simulink model "KD_cl_harness_cl_ouports_added"  (R2015b)
settings: Solver=ode45  StartTime=0  StopTime=inf  FixedStep=0.01  MaxStep=0.005  RelTol=1e-5  AbsTol=1e-5
undefined symbols (not defined in the file or in its folder): A2, bin_vec, c_0, c_1000, c_1000inv, c_100inv, c_1d2p4, c_1p7, c_4400inv, c_5500inv, c_80, c_compmap, c_ctok, c_fflow_max, c_fflow_min, c_filt, c_flowdiv, c_flowmin, c_flowmult, c_inf, c_km1d2k, c_n1, c_p00001, c_p01, c_p1e9, c_p4d1p4, c_pincomp, c_rair, c_roacorr, c_rpmtoradpers, c_svrthrottle1, c_svrthrottle2, c_svrthrottlearg, c_svrthrottlebeta, c_vnliftmax, c_vnliftmin, cl_offset, clff, Coefs, const, const_exhat, const_vec, Dual_array, dual_zero, egr_ecu_ff, expcon, f_mat, gs_jul, HQP_eps, HQP_INF, HQP_saturation, IV, L2, length_L, maxL, mHQP_saturation, minL, Newton, nRed, num_constraints ... (+22)
libraries: simulink x33
(part 5 of 6)

== system KD_cl_harness_cl_ouports_added/ctrl_rb_explicit_20140220_v6_simp/ntremap/remap_wt_to_map/ThrottleModel1/AirModel_map_use ==
  TA_deg : Inport
  Ne_rpm : Inport  Port=2
  Pim_Pa : Inport  Port=3
  Ta_K : Inport  Port=4
  R_a : Inport  Port=5
  wegrthr : Inport  Port=6
  Forward_Flow : Subsystem
  Product1 : Product  Inputs=*//  SaturateOnIntegerOverflow=on  RndMeth=Zero  InputSameDT=on  OutDataTypeStr=Inherit: Same as first input
  Saturation1 : Saturate  UpperLimit=c_inf  LowerLimit=c_p1e9
      settings: AttributesFormatString=%<LowerLimit>\n%<UpperLimit>
  Saturation5 : Saturate  UpperLimit=c_inf  LowerLimit=c_p1e9
      settings: AttributesFormatString=%<LowerLimit>\n%<UpperLimit>
  one : Constant  OutDataTypeStr=single  SampleTime=-1
      settings: AttributesFormatString=%<Value>\n%<SampleTime>
  p_pre_throttle : Outport
  sat_out-45 : Outport  Port=2
  sat_out-46 : Outport  Port=3
  sat_out-58 : Outport  Port=4
  sat_out-59 : Outport  Port=5
  sat_out-60 : Outport  Port=6
  sat_out-61 : Outport  Port=7
  sat_out-62 : Outport  Port=8
  sat_out-63 : Outport  Port=9
  sat_out-64 : Outport  Port=10
  sat_out-65 : Outport  Port=11
  out-17 : Outport  Port=12
  out-28 : Outport  Port=13
  wires:
  Saturation1/1 -> Product1/3
  Saturation5/1 -> Product1/2
  Forward_Flow/1(p_pre_throttle) -> p_pre_throttle/1
  wegrthr/1 -> Forward_Flow/5(wegrthr)
  Ne_rpm/1 -> Forward_Flow/3(Ne_rpm)
  one/1 -> Product1/1
  R_a/1 -> Saturation1/1, sat_out-45/1
  Ta_K/1 -> Saturation5/1, sat_out-46/1
  Pim_Pa/1 -> Forward_Flow/4(Pm)
  TA_deg/1 -> Forward_Flow/2(TA_deg)
  Product1/1 -> Forward_Flow/1(Ro_a)
  Forward_Flow/2(sat_out-58) -> sat_out-58/1
  Forward_Flow/3(sat_out-59) -> sat_out-59/1
  Forward_Flow/4(sat_out-60) -> sat_out-60/1
  Forward_Flow/5(sat_out-61) -> sat_out-61/1
  Forward_Flow/6(sat_out-62) -> sat_out-62/1
  Forward_Flow/7(sat_out-63) -> sat_out-63/1
  Forward_Flow/8(sat_out-64) -> sat_out-64/1
  Forward_Flow/9(sat_out-65) -> sat_out-65/1
  Forward_Flow/10(out-17) -> out-17/1
  Forward_Flow/11(out-28) -> out-28/1

== system KD_cl_harness_cl_ouports_added/ctrl_rb_explicit_20140220_v6_simp/pex_estimator/WhileIteratorSubsystem/newton/For_Iterator_Subsystem ==
  u : Inport
  sv1 : Inport  Port=2
  sv2 : Inport  Port=3
  arg : Inport  Port=4
  beta : Inport  Port=5
  Demux : Demux  Outputs=2
  Divide : Product  Inputs=*/
  For Iterator : ForIterator  ResetStates=reset  IterationLimit=SVR_EGR_exhat.num_SV
  Gain : Gain  Gain=100
      settings: AttributesFormatString=%<Gain>
  Product{,1..3} (4 alike) : Product  RndMeth=Zero
  Saturation1 : Saturate  UpperLimit=9  LowerLimit=1
      settings: AttributesFormatString=%<LowerLimit>\n%<UpperLimit>
  Selector : Selector  InputPortWidth=SVR_EGR_exhat.num_SV  IndexOptions=Index vector (port)  Indices=[1 3]  OutputSizes=1
  Selector1 : Selector  InputPortWidth=SVR_EGR_exhat.num_SV  IndexOptions=Index vector (port)  Indices=[1 3]  OutputSizes=1
  Selector2 : Selector  InputPortWidth=SVR_EGR_exhat.num_SV  IndexOptions=Index vector (port)  Indices=[1 3]  OutputSizes=1
  Sum : Sum  Inputs=|-+
  Sum1 : Sum  Inputs=+-|
  Sum2 : Sum  Inputs=-|-
  Sum3 : Sum  Inputs=++|
  Unit Delay : UnitDelay  SampleTime=-1
  exp Lookup Table : Lookup  InputValues=SVR_EGR_exhat.exp.x  Table=SVR_EGR_exhat.exp.y  LookUpMeth=Interpolation-Use End Values
      settings: AttributesFormatString=%<LookUpMeth>\n%<InputValues>
  ba : Outport  OutDataTypeStr=single
  sat_out-47 : Outport  Port=2
  wires:
  Saturation1/1 -> [iter]
  For Iterator/1 -> Saturation1/1, sat_out-47/1
  [iter] -> Selector2/2
  [iter] -> Selector1/2
  [iter] -> Selector/2
  Sum3/1 -> ba/1, Unit Delay/1
  Product3/1 -> Sum3/2
  Selector2/1 -> Product3/2
  Gain/1 -> Divide/2
  Product2/1 -> Gain/1
  arg/1 -> Product2/2, Product2/1
  Sum2/1 -> Divide/1
  Product1/1 -> Sum2/2
  Product/1 -> Sum2/1
  Sum1/1 -> Product1/2, Product1/1
  Sum/1 -> Product/2, Product/1
  Demux/2 -> Sum1/1
  Selector1/1 -> Sum1/2
  Demux/1 -> Sum/2
  Selector/1 -> Sum/1
  u/1 -> Demux/1
  beta/1 -> Selector2/1
  sv2/1 -> Selector1/1
  sv1/1 -> Selector/1
  Unit Delay/1 -> Sum3/1
  Divide/1 -> exp Lookup Table/1
  exp Lookup Table/1 -> Product3/1

== system KD_cl_harness_cl_ouports_added/ctrl_rb_explicit_20140220_v6_simp/pex_estimator/WhileIteratorSubsystem/newton/If_Action_Subsystem ==
  pex : Inport
  ba : Inport  Port=2
  c : Inport  Port=3
  k : Inport  Port=4
  Action Port : ActionPort  ActionType=then
  Gain1 : Gain  Gain=2
  Gain6 : Gain  Gain=2
  Mux : Mux  Inputs=2
  Product : Product  Inputs=***  RndMeth=Zero
  Product1 : Product  Inputs=*/  RndMeth=Zero
  Product2 : Product  Inputs=**  RndMeth=Zero
  Product3 : Product  Inputs=***  RndMeth=Zero
  Product4 : Product  Inputs=*/  RndMeth=Zero
  Saturation1 : Saturate  UpperLimit=inf  LowerLimit=0
      settings: AttributesFormatString=%<LowerLimit>\n%<UpperLimit>
  Saturation2 : Saturate  UpperLimit=inf  LowerLimit=0
      settings: AttributesFormatString=%<LowerLimit>\n%<UpperLimit>
  Saturation3 : Saturate  UpperLimit=c_inf  LowerLimit=c_p1e9
      settings: AttributesFormatString=%<LowerLimit>\n%<UpperLimit>
  Saturation4 : Saturate  UpperLimit=c_inf  LowerLimit=c_p1e9
      settings: AttributesFormatString=%<LowerLimit>\n%<UpperLimit>
  Sqrt1 : Sqrt  AlgorithmType=Newton-Raphson  SaturateOnIntegerOverflow=on
  Sqrt2 : Sqrt  AlgorithmType=Newton-Raphson  SaturateOnIntegerOverflow=on
  Sum1 : Sum  Inputs=++|
  Sum3 : Sum  Inputs=++|
  one : Constant  OutDataTypeStr=single  SampleTime=-1
      settings: AttributesFormatString=%<Value>\n%<SampleTime>
  one1 : Constant  OutDataTypeStr=single  SampleTime=-1
      settings: AttributesFormatString=%<Value>\n%<SampleTime>
  Out : Outport
  sat_out-48 : Outport  Port=2
  sat_out-49 : Outport  Port=3
  sat_out-50 : Outport  Port=4
  sat_out-51 : Outport  Port=5
  wires:
  Saturation4/1 -> Product4/2
  Saturation3/1 -> Product1/2
  Saturation2/1 -> Sqrt1/1
  Saturation1/1 -> Sqrt2/1
  Product3/1 -> Product2/1
  Sqrt1/1 -> Product3/3
  Product4/1 -> Saturation2/1, sat_out-49/1
  Gain1/1 -> Saturation4/1, sat_out-51/1
  Sum1/1 -> Gain1/1
  one1/1 -> Sum1/1
  [k] -> Sum1/2
  [k] -> Product4/1
  [c] -> Product3/2
  [ba] -> Product3/1
  Mux/1 -> Out/1
  Product2/1 -> Mux/2
  Product/1 -> Mux/1
  Sqrt2/1 -> Product/3
  [pex] -> Product2/2
  Product1/1 -> Saturation1/1, sat_out-48/1
  Gain6/1 -> Saturation3/1, sat_out-50/1
  Sum3/1 -> Gain6/1
  one/1 -> Sum3/1
  [k] -> Sum3/2
  [k] -> Product1/1
  [c] -> Product/2
  [ba] -> Product/1
  k/1 -> [k]
  pex/1 -> [pex]
  c/1 -> [c]
  ba/1 -> [ba]

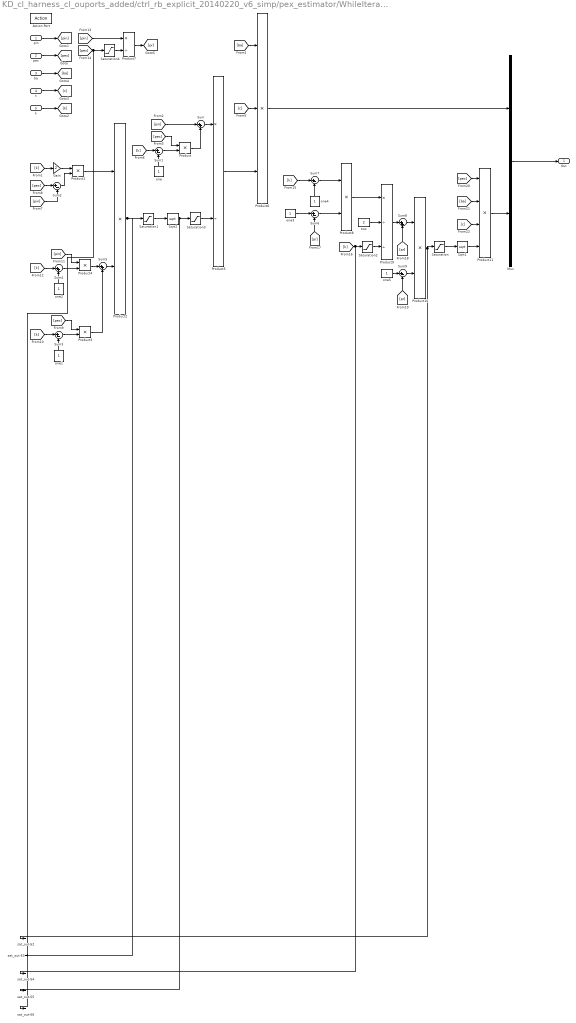
== system KD_cl_harness_cl_ouports_added/ctrl_rb_explicit_20140220_v6_simp/pex_estimator/WhileIteratorSubsystem/newton/If_Action_Subsystem1 ==
  pin : Inport
  pex : Inport  Port=2
  ba : Inport  Port=3
  c : Inport  Port=4
  k : Inport  Port=5
  Action Port : ActionPort  ActionType=else
  Gain : Gain  Gain=2
  Mux : Mux  Inputs=2
  Product{,1..4} (5 alike) : Product  RndMeth=Zero
  Product10 : Product  Inputs=**  RndMeth=Zero
  Product11 : Product  Inputs=****  RndMeth=Zero
  Product5 : Product  Inputs=*/  RndMeth=Zero
  Product6 : Product  Inputs=***  RndMeth=Zero
  Product7 : Product  Inputs=*/  RndMeth=Zero
  Product8 : Product  Inputs=**  RndMeth=Zero
  Product9 : Product  Inputs=*//  RndMeth=Zero
  Saturation : Saturate  UpperLimit=inf  LowerLimit=0
      settings: AttributesFormatString=%<LowerLimit>\n%<UpperLimit>
  Saturation1 : Saturate  UpperLimit=inf  LowerLimit=0
      settings: AttributesFormatString=%<LowerLimit>\n%<UpperLimit>
  Saturation2 : Saturate  UpperLimit=c_inf  LowerLimit=c_p1e9
      settings: AttributesFormatString=%<LowerLimit>\n%<UpperLimit>
  Saturation3 : Saturate  UpperLimit=c_inf  LowerLimit=c_p00001
      settings: AttributesFormatString=%<LowerLimit>\n%<UpperLimit>
  Saturation4 : Saturate  UpperLimit=c_inf  LowerLimit=c_p1e9
      settings: AttributesFormatString=%<LowerLimit>\n%<UpperLimit>
  Sqrt1 : Sqrt  AlgorithmType=Newton-Raphson  SaturateOnIntegerOverflow=on
  Sqrt2 : Sqrt  AlgorithmType=Newton-Raphson  SaturateOnIntegerOverflow=on
  Sum{,4..5,8} (4 alike) : Sum  Inputs=|++
  Sum{1..3,6..7,9} (6 alike) : Sum  Inputs=|+-
  one{,1..5} (6 alike) : Constant  OutDataTypeStr=single  SampleTime=-1
      settings: AttributesFormatString=%<Value>\n%<SampleTime>
  two : Constant  Value=2  OutDataTypeStr=single  SampleTime=-1
      settings: AttributesFormatString=%<Value>\n%<SampleTime>
  Out : Outport
  sat_out-52 : Outport  Port=2
  sat_out-53 : Outport  Port=3
  sat_out-54 : Outport  Port=4
  sat_out-55 : Outport  Port=5
  sat_out-56 : Outport  Port=6
  wires:
  Saturation4/1 -> Product7/2
  Saturation2/1 -> Product9/3
  Saturation1/1 -> Sqrt2/1
  Saturation/1 -> Sqrt1/1
  Mux/1 -> Out/1
  Product6/1 -> Mux/1
  Product11/1 -> Mux/2
  [c] -> Product11/3
  [ba] -> Product11/2
  [pex] -> Product11/1
  Sqrt1/1 -> Product11/4
  Product10/1 -> Saturation/1, sat_out-52/1
  Sum8/1 -> Product10/1
  [pr] -> Sum9/2
  Sum9/1 -> Product10/2
  one5/1 -> Sum9/1
  [pr] -> Sum8/2
  Product9/1 -> Sum8/1
  [pr] -> Sum6/2
  Product7/1 -> [pr]
  [k] -> Saturation2/1, sat_out-54/1
  two/1 -> Product9/2
  Product8/1 -> Product9/1
  Sum7/1 -> Product8/1
  Sum6/1 -> Product8/2
  one4/1 -> Sum7/2
  [k] -> Sum7/1
  [pex] -> Saturation4/1, sat_out-56/1
  [pin] -> Product7/1
  one3/1 -> Sum6/1
  Product5/1 -> Product6/3
  [c] -> Product6/2
  [ba] -> Product6/1
  Sum/1 -> Product5/1
  Sqrt2/1 -> Saturation3/1, sat_out-55/1
  Product2/1 -> Saturation1/1, sat_out-53/1
  Product3/1 -> Sum5/2
  Product4/1 -> Sum5/1
  Sum5/1 -> Product2/2
  [pin] -> Product4/1
  Sum4/1 -> Product4/2
  [k] -> Sum4/1
  one2/1 -> Sum4/2
  [pex] -> Product3/1
  Sum3/1 -> Product3/2
  [k] -> Sum3/1
  one1/1 -> Sum3/2
  Product1/1 -> Product2/1
  Gain/1 -> Product1/1
  Sum2/1 -> Product1/2
  [pex] -> Sum2/1
  [pin] -> Sum2/2
  [k] -> Gain/1
  Product/1 -> Sum/2
  [pex] -> Product/1
  Sum1/1 -> Product/2
  [k] -> Sum1/1
  one/1 -> Sum1/2
  [pin] -> Sum/1
  pin/1 -> [pin]
  k/1 -> [k]
  c/1 -> [c]
  ba/1 -> [ba]
  pex/1 -> [pex]
  Saturation3/1 -> Product5/2

== system KD_cl_harness_cl_ouports_added/ctrl_rb_explicit_20140220_v6_simp/pex_estimator/WhileIteratorSubsystem/newton/If_Action_Subsystem2 ==
  pex_hat : Inport
  Action Port : ActionPort  ActionType=else
  pex : Outport
  wires:
  pex_hat/1 -> pex/1

== system KD_cl_harness_cl_ouports_added/ctrl_rb_explicit_20140220_v6_simp/pex_estimator/WhileIteratorSubsystem/newton/If_Action_Subsystem3 ==
  valve : Inport
  pex_hat : Inport  Port=2
  pex_ecu : Inport  Port=3
  Action Port : ActionPort  ActionType=then
  Divide : Product  Inputs=*/
  Divide1 : Product  Inputs=**
  Divide2 : Product  Inputs=**
  Sum : Sum  Inputs=-+|
  Sum1 : Sum  Inputs=+|+
  fifteen : Constant  Value=15  OutDataTypeStr=single  SampleTime=-1
      settings: AttributesFormatString=%<Value>\n%<SampleTime>
  one : Constant  OutDataTypeStr=single  SampleTime=-1
      settings: AttributesFormatString=%<Value>\n%<SampleTime>
  pex : Outport
  wires:
  valve/1 -> Divide/1
  fifteen/1 -> Divide/2
  Divide/1 -> Divide1/2, Sum/1
  pex_hat/1 -> Divide1/1
  one/1 -> Sum/2
  Sum/1 -> Divide2/1
  pex_ecu/1 -> Divide2/2
  Divide1/1 -> Sum1/1
  Divide2/1 -> Sum1/2
  Sum1/1 -> pex/1

== system KD_cl_harness_cl_ouports_added/ctrl_rb_explicit_20140220_v6_simp/pex_estimator/WhileIteratorSubsystem/newton/update ==
  dwdp : Inport
  error : Inport  Port=2
  Data Store Read11 : DataStoreRead  DataStoreName=man_pex_eps
  Product2 : Product  Inputs=**  RndMeth=Zero
  Product8 : Product  Inputs=/**  RndMeth=Zero
  Saturation3 : Saturate  UpperLimit=c_inf  LowerLimit=c_p1e9
      settings: AttributesFormatString=%<LowerLimit>\n%<UpperLimit>
  Sum2 : Sum  Inputs=|++
  man_pex_eps : Gain
  delta : Outport
  sat_out-57 : Outport  Port=2
  wires:
  Data Store Read11/1 -> man_pex_eps/1
  Sum2/1 -> Saturation3/1, sat_out-57/1
  Saturation3/1 -> Product8/1
  Product2/1 -> Sum2/2
  error/1 -> Product8/3
  dwdp/1 -> Product2/1, Product8/2, Product2/2
  Product8/1 -> delta/1
  man_pex_eps/1 -> Sum2/1

== system KD_cl_harness_cl_ouports_added/EGR Throttle/EGR Throttle/Throttle Model2/Air Model_map_use/Back-Flow/Cal phi1 ==
  Pm : Inport
  Ro_m : Inport  Port=2
  Gain2 : Gain  Gain=1/(const.Pcab*const.Pcab/const.Rair/const.Tcab)  SaturateOnIntegerOverflow=on  OutDataTypeStr=Inherit: Same as input  ParamDataTypeStr=Inherit: Same as input
  Math Function : Sqrt  Operator=signedSqrt  AlgorithmType=Newton-Raphson  SaturateOnIntegerOverflow=on
  Product4 : Product  Inputs=**  SaturateOnIntegerOverflow=on  RndMeth=Zero  InputSameDT=on  OutDataTypeStr=Inherit: Same as first input
  phi : Outport
  wires:
  Math Function/1 -> phi/1
  Ro_m/1 -> Product4/2
  Pm/1 -> Product4/1
  Gain2/1 -> Math Function/1
  Product4/1 -> Gain2/1

== system KD_cl_harness_cl_ouports_added/EGR Throttle/EGR Throttle/Throttle Model2/Air Model_map_use/Forward-Flow/Cal phi ==
  Pa : Inport
  Ro_a : Inport  Port=2
  Gain2 : Gain  Gain=1/(const.Pcab*const.Pcab/const.Rair/const.Tcab)  SaturateOnIntegerOverflow=on  OutDataTypeStr=Inherit: Same as input  ParamDataTypeStr=Inherit: Same as input
  Math Function : Sqrt  Operator=signedSqrt  AlgorithmType=Newton-Raphson  SaturateOnIntegerOverflow=on
  Product4 : Product  Inputs=**  SaturateOnIntegerOverflow=on  RndMeth=Zero  InputSameDT=on  OutDataTypeStr=Inherit: Same as first input
  phi : Outport
  wires:
  Math Function/1 -> phi/1
  Ro_a/1 -> Product4/2
  Pa/1 -> Product4/1
  Gain2/1 -> Math Function/1
  Product4/1 -> Gain2/1

== system KD_cl_harness_cl_ouports_added/EGR Valve/SVR EGR/EGR_model/Air Model_map_use/Back-Flow/Cal phi1 ==
  Pm : Inport
  Ro_m : Inport  Port=2
  Gain2 : Gain  Gain=1/(const.Pcab*const.Pcab/const.Rair/const.Tcab)  SaturateOnIntegerOverflow=on  OutDataTypeStr=Inherit: Same as input  ParamDataTypeStr=Inherit: Same as input
  Math Function : Sqrt  Operator=signedSqrt  AlgorithmType=Newton-Raphson  SaturateOnIntegerOverflow=on
  Product4 : Product  Inputs=**  SaturateOnIntegerOverflow=on  RndMeth=Zero  InputSameDT=on  OutDataTypeStr=Inherit: Same as first input
  phi : Outport
  wires:
  Product4/1 -> Gain2/1
  Gain2/1 -> Math Function/1
  Pm/1 -> Product4/1
  Ro_m/1 -> Product4/2
  Math Function/1 -> phi/1

== system KD_cl_harness_cl_ouports_added/EGR Valve/SVR EGR/EGR_model/Air Model_map_use/Forward-Flow/Cal phi ==
  Pa : Inport
  Ro_a : Inport  Port=2
  Gain2 : Gain  Gain=1/(const.Pcab*const.Pcab/const.Rair/const.Tcab)  SaturateOnIntegerOverflow=on  OutDataTypeStr=Inherit: Same as input  ParamDataTypeStr=Inherit: Same as input
  Math Function : Sqrt  Operator=signedSqrt  AlgorithmType=Newton-Raphson  SaturateOnIntegerOverflow=on
  Product4 : Product  Inputs=**  SaturateOnIntegerOverflow=on  RndMeth=Zero  InputSameDT=on  OutDataTypeStr=Inherit: Same as first input
  phi : Outport
  wires:
  Product4/1 -> Gain2/1
  Gain2/1 -> Math Function/1
  Pa/1 -> Product4/1
  Ro_a/1 -> Product4/2
  Math Function/1 -> phi/1

== system KD_cl_harness_cl_ouports_added/ctrl_rb_explicit_20140220_v6_simp/HQPKWIK_V6/QPKWIK_Main/QPKWIK_While_Loop/Case1/Continue ==
  Continue : ActionPort  ActionType=else
  Constant : Constant  Value=2  OutDataTypeStr=uint8
  Run : Outport  InitialOutput=2
  wires:
  Constant/1 -> Run/1

== system KD_cl_harness_cl_ouports_added/ctrl_rb_explicit_20140220_v6_simp/HQPKWIK_V6/QPKWIK_Main/QPKWIK_While_Loop/Case1/Stop ==
  Stop : ActionPort  ActionType=then
  Constant : Constant  Value=5  OutDataTypeStr=uint8
  Run : Outport  InitialOutput=5
  wires:
  Constant/1 -> Run/1

== system KD_cl_harness_cl_ouports_added/ctrl_rb_explicit_20140220_v6_simp/HQPKWIK_V6/QPKWIK_Main/QPKWIK_While_Loop/Case1/Stop1 ==
  Stop : ActionPort  ActionType=elseif
  Constant : Constant  Value=5  OutDataTypeStr=uint8
  Run : Outport  InitialOutput=5
  wires:
  Constant/1 -> Run/1

== system KD_cl_harness_cl_ouports_added/ctrl_rb_explicit_20140220_v6_simp/HQPKWIK_V6/QPKWIK_Main/QPKWIK_While_Loop/Case2/Dual_direction ==
  Dual_array : Inport
  Aknext : Inport  Port=2
  Dual_direction : ActionPort  ActionType=then
  Product : Product  Multiplication=Matrix(*)  RndMeth=Zero
  r : Outport  InitialOutput=zero_vec
  wires:
  Product/1 -> r/1
  Aknext/1 -> Product/2
  Dual_array/1 -> Product/1

== system KD_cl_harness_cl_ouports_added/ctrl_rb_explicit_20140220_v6_simp/HQPKWIK_V6/QPKWIK_Main/QPKWIK_While_Loop/Case2/Nominal_dual_direction ==
  Nominal_dual_direction : ActionPort  ActionType=else
  zeros : Constant  Value=zero_vec  VectorParams1D=off  OutDataTypeStr=single
      settings: AttributesFormatString=%<VectorParams1D>
  r : Outport  InitialOutput=zero_vec
  wires:
  zeros/1 -> r/1

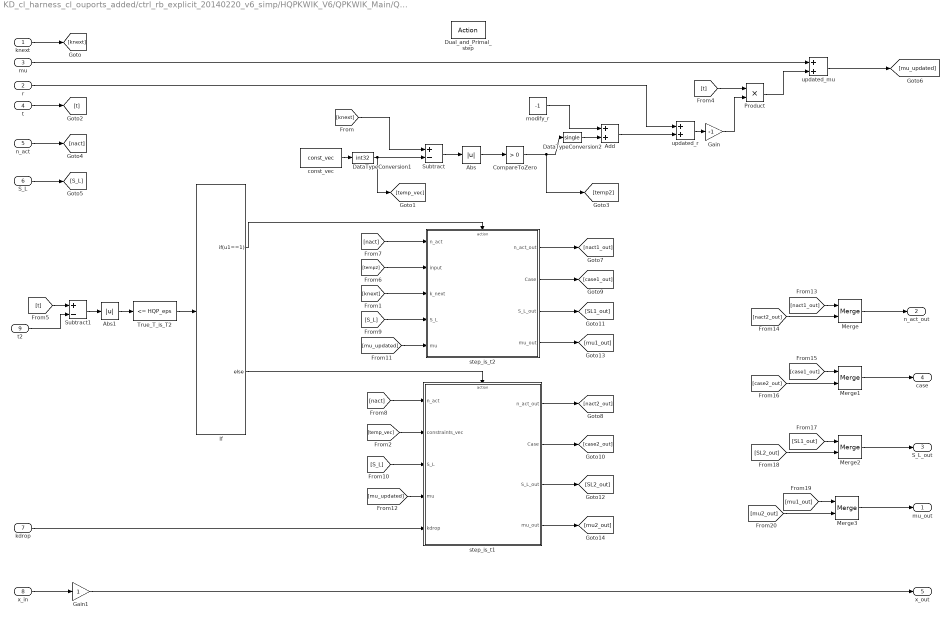
== system KD_cl_harness_cl_ouports_added/ctrl_rb_explicit_20140220_v6_simp/HQPKWIK_V6/QPKWIK_Main/QPKWIK_While_Loop/Case3/Dual_and_Primal_step ==
  knext : Inport
  r : Inport  Port=2
  mu : Inport  Port=3
  t : Inport  Port=4
  n_act : Inport  Port=5
  S_L : Inport  Port=6
  kdrop : Inport  Port=7
  x_in : Inport  Port=8
  t2 : Inport  Port=9
  Dual_and_Primal_step : ActionPort  ActionType=else
  Abs : Abs  SaturateOnIntegerOverflow=on
  Abs1 : Abs
  Add : Sum
  CompareToZero : simulink/Logic and Bit Operations/Compare To Zero  relop=>  OutDataTypeStr=boolean
  DataTypeConversion1 : DataTypeConversion  OutDataTypeStr=int32
  DataTypeConversion2 : DataTypeConversion  OutDataTypeStr=single
  Gain : Gain  Gain=-1
  Gain1 : Gain
  If : If  IfExpression=u1==1
  Merge{,1..3} (4 alike) : Merge
  Product : Product  RndMeth=Zero
  Subtract : Sum  Inputs=+-
  Subtract1 : Sum  Inputs=+-
  True_T_is_T2 : simulink/Logic and Bit Operations/Compare To Constant  relop=<=  const=HQP_eps  OutDataTypeStr=boolean
  const_vec : Constant  Value=const_vec  VectorParams1D=off  OutDataTypeStr=single
      settings: AttributesFormatString=%<VectorParams1D>
  modify_r : Constant  Value=-1  OutDataTypeStr=single
  step_is_t1 : Subsystem  TreatAsAtomicUnit=on
  step_is_t2 : Subsystem  TreatAsAtomicUnit=on
  updated_mu : Sum
  updated_r : Sum
  mu_out : Outport  InitialOutput=zero_vec
  n_act_out : Outport  Port=2  InitialOutput=0
  S_L_out : Outport  Port=3  InitialOutput=zero_vec
  case : Outport  Port=4  InitialOutput=1
  x_out : Outport  Port=5  InitialOutput=ov_zero_vec
  wires:
  Product/1 -> updated_mu/2
  Abs1/1 -> True_T_is_T2/1
  t2/1 -> Subtract1/2
  [t] -> Subtract1/1
  Subtract1/1 -> Abs1/1
  True_T_is_T2/1 -> If/1
  DataTypeConversion2/1 -> Add/2
  DataTypeConversion1/1 -> [temp_vec], Subtract/2
  Gain1/1 -> x_out/1
  x_in/1 -> Gain1/1
  kdrop/1 -> step_is_t1/5(kdrop)
  Merge1/1 -> case/1
  Merge3/1 -> mu_out/1
  Merge2/1 -> S_L_out/1
  Merge/1 -> n_act_out/1
  If/2 -> step_is_t1/Action
  If/1 -> step_is_t2/Action
  const_vec/1 -> DataTypeConversion1/1
  modify_r/1 -> Add/1
  Add/1 -> updated_r/2
  r/1 -> updated_r/1
  mu/1 -> updated_mu/1
  updated_r/1 -> Gain/1
  Gain/1 -> Product/2
  knext/1 -> [knext]
  [knext] -> Subtract/1
  [knext] -> step_is_t2/3(k_next)
  [temp_vec] -> step_is_t1/2(constraints_vec)
  t/1 -> [t]
  [t] -> Product/1
  [temp2] -> step_is_t2/2(input)
  n_act/1 -> [nact]
  [nact] -> step_is_t2/1(n_act)
  [nact] -> step_is_t1/1(n_act)
  S_L/1 -> [S_L]
  [S_L] -> step_is_t2/4(S_L)
  [S_L] -> step_is_t1/3(S_L)
  updated_mu/1 -> [mu_updated]
  [mu_updated] -> step_is_t2/5(mu)
  [mu_updated] -> step_is_t1/4(mu)
  step_is_t2/1(n_act_out) -> [nact1_out]
  step_is_t1/1(n_act_out) -> [nact2_out]
  step_is_t2/2(Case) -> [case1_out]
  step_is_t1/2(Case) -> [case2_out]
  step_is_t2/3(S_L_out) -> [SL1_out]
  step_is_t1/3(S_L_out) -> [SL2_out]
  step_is_t2/4(mu_out) -> [mu1_out]
  step_is_t1/4(mu_out) -> [mu2_out]
  [nact1_out] -> Merge/1
  [nact2_out] -> Merge/2
  [case1_out] -> Merge1/1
  [case2_out] -> Merge1/2
  [SL1_out] -> Merge2/1
  [SL2_out] -> Merge2/2
  [mu1_out] -> Merge3/1
  [mu2_out] -> Merge3/2
  Subtract/1 -> Abs/1
  Abs/1 -> CompareToZero/1
  CompareToZero/1 -> DataTypeConversion2/1, [temp2]

== system KD_cl_harness_cl_ouports_added/ctrl_rb_explicit_20140220_v6_simp/HQPKWIK_V6/QPKWIK_Main/QPKWIK_While_Loop/Case3/Dual_step ==
  n_act : Inport
  constraints_vec : Inport  Port=2
  S_L : Inport  Port=3
  mu : Inport  Port=4
  kdrop : Inport  Port=5
  knext : Inport  Port=6
  r : Inport  Port=7
  t : Inport  Port=8
  x_in : Inport  Port=9
  Dual_step : ActionPort  ActionType=elseif
  Abs : Abs  SaturateOnIntegerOverflow=on
  Abs1 : Abs  SaturateOnIntegerOverflow=on
  Add : Sum
  CompareToZero : simulink/Logic and Bit Operations/Compare To Zero  relop=>  OutDataTypeStr=boolean
  CompareToZero1 : simulink/Logic and Bit Operations/Compare To Zero  relop=>  OutDataTypeStr=boolean
  Constant2 : Constant  Value=2  OutDataTypeStr=uint8
  DataTypeConversion1 : DataTypeConversion  OutDataTypeStr=int32
  DataTypeConversion2 : DataTypeConversion  OutDataTypeStr=single
  DataTypeConversion3 : DataTypeConversion  OutDataTypeStr=single
  DataTypeConversion4 : DataTypeConversion  OutDataTypeStr=int32
  Gain : Gain  Gain=-1
  Gain1 : Gain
  Product : Product  RndMeth=Zero
  Product1 : Product  OutDataTypeStr=int32  RndMeth=Zero
  Product2 : Product  OutDataTypeStr=single  RndMeth=Zero
  Subtract : Sum  Inputs=+-
  Subtract1 : Sum  Inputs=+-
  add : Sum  OutDataTypeStr=int32
  add1 : Sum
  add2 : Sum
  reduce_num_constraints : Constant  Value=-1  OutDataTypeStr=int32
  update_r : Constant  Value=-1  OutDataTypeStr=single
  n_act_out : Outport  InitialOutput=0
  Case : Outport  Port=2  InitialOutput=2
  S_L_out : Outport  Port=3  InitialOutput=zero_vec
  mu_out : Outport  Port=4  InitialOutput=zero_vec
  x_out : Outport  Port=5  InitialOutput=ov_zero_vec
  wires:
  DataTypeConversion4/1 -> Product1/1, DataTypeConversion3/1
  DataTypeConversion1/1 -> Subtract/2, Subtract1/2
  DataTypeConversion3/1 -> Product2/1
  DataTypeConversion2/1 -> Add/2
  Gain1/1 -> x_out/1
  x_in/1 -> Gain1/1
  add1/1 -> Product2/2
  t/1 -> Product/1
  constraints_vec/1 -> DataTypeConversion1/1
  update_r/1 -> Add/1
  Add/1 -> add2/2
  knext/1 -> Subtract1/1
  r/1 -> add2/1
  mu/1 -> add1/1
  add2/1 -> Gain/1
  Gain/1 -> Product/2
  Product/1 -> add1/2
  CompareToZero/1 -> DataTypeConversion4/1
  kdrop/1 -> Subtract/1
  reduce_num_constraints/1 -> add/1
  n_act/1 -> add/2
  add/1 -> n_act_out/1
  Constant2/1 -> Case/1
  S_L/1 -> Product1/2
  Product1/1 -> S_L_out/1
  Product2/1 -> mu_out/1
  Subtract/1 -> Abs/1
  Abs/1 -> CompareToZero/1
  Subtract1/1 -> Abs1/1
  Abs1/1 -> CompareToZero1/1
  CompareToZero1/1 -> DataTypeConversion2/1

== system KD_cl_harness_cl_ouports_added/ctrl_rb_explicit_20140220_v6_simp/HQPKWIK_V6/QPKWIK_Main/QPKWIK_While_Loop/Case3/Infeasible ==
  x0 : Inport
  Infeasible : ActionPort  ActionType=then
  stop_run : Constant  Value=5  OutDataTypeStr=uint8
  run1 : Outport  InitialOutput=5
  x_infeas : Outport  Port=2  InitialOutput=ov_zero_vec
  wires:
  stop_run/1 -> run1/1
  x0/1 -> x_infeas/1

== system KD_cl_harness_cl_ouports_added/ctrl_rb_explicit_20140220_v6_simp/HQPKWIK_V6/QPKWIK_Main/QPKWIK_While_Loop/Case3/Infinite_t2 ==
  Infinite_t2 : ActionPort  ActionType=then
  infinity : Constant  Value=HQP_INF  OutDataTypeStr=single
  t2 : Outport  InitialOutput=HQP_INF
  wires:
  infinity/1 -> t2/1

== system KD_cl_harness_cl_ouports_added/ctrl_rb_explicit_20140220_v6_simp/HQPKWIK_V6/QPKWIK_Main/QPKWIK_While_Loop/Case3/Max_number_in_SL ==
  Max_number_in_SL : ActionPort  ActionType=elseif
  infinity : Constant  Value=HQP_INF  OutDataTypeStr=single
  t1 : Outport  InitialOutput=HQP_INF
  wires:
  infinity/1 -> t1/1

== system KD_cl_harness_cl_ouports_added/ctrl_rb_explicit_20140220_v6_simp/HQPKWIK_V6/QPKWIK_Main/QPKWIK_While_Loop/Case3/Nominal_dual_length ==
  Nominal_dual_step : ActionPort  ActionType=then
  infinity : Constant  Value=HQP_INF  OutDataTypeStr=single
  t1 : Outport  InitialOutput=HQP_INF
  wires:
  infinity/1 -> t1/1

== system KD_cl_harness_cl_ouports_added/ctrl_rb_explicit_20140220_v6_simp/HQPKWIK_V6/QPKWIK_Main/QPKWIK_While_Loop/Case3/T1_calculation ==
  mu : Inport
  r : Inport  Port=2
  contraints_vec : Inport  Port=3
  INF : Inport  Port=4
  T1_calculation : ActionPort  ActionType=else
  Abs : Abs
  Abs1 : Abs
  CompareToConstant : simulink/Logic and Bit Operations/Compare To Constant  relop=<=  const=HQP_eps  OutDataTypeStr=boolean
  CompareToConstant1 : simulink/Logic and Bit Operations/Compare To Constant  relop=<=  const=HQP_eps  OutDataTypeStr=boolean
  CompareToZero2 : simulink/Logic and Bit Operations/Compare To Zero  relop=>  OutDataTypeStr=boolean
  DataTypeConversion1 : DataTypeConversion  OutDataTypeStr=int32
  DataTypeConversion2 : DataTypeConversion  OutDataTypeStr=int32
  DataTypeConversion3 : DataTypeConversion  OutDataTypeStr=single
  DataTypeConversion4 : DataTypeConversion  OutDataTypeStr=single
  Divide : Product  Inputs=*/
  MinMax : MinMax
  MinMax1 : MinMax
  Product1 : Product  RndMeth=Zero
  Product2 : Product  Multiplication=Matrix(*)  OutDataTypeStr=int32  RndMeth=Zero
  Product4 : Product  RndMeth=Zero
  Subtract : Sum  Inputs=+-
  Zero_protection : Subsystem
  add : Sum
  transpose : Math  Operator=transpose  SaturateOnIntegerOverflow=on
  kdrop : Outport  InitialOutput=0
  t1 : Outport  Port=2  InitialOutput=0
  wires:
  DataTypeConversion4/1 -> Zero_protection/1(In2), Product4/1
  DataTypeConversion3/1 -> Product1/1
  CompareToConstant/1 -> DataTypeConversion3/1
  DataTypeConversion2/1 -> Product2/1
  DataTypeConversion1/1 -> Product2/2
  Product4/1 -> add/1, Subtract/1, Abs/1
  CompareToZero2/1 -> DataTypeConversion4/1
  INF/1 -> Product1/2
  Abs/1 -> CompareToConstant/1
  MinMax1/1 -> t1/1
  transpose/1 -> DataTypeConversion2/1
  contraints_vec/1 -> transpose/1
  CompareToConstant1/1 -> DataTypeConversion1/1
  Product2/1 -> kdrop/1
  r/1 -> [r], Zero_protection/2(In1), CompareToZero2/1
  Divide/1 -> Product4/2
  mu/1 -> Divide/1
  add/1 -> MinMax1/1, MinMax/1
  Product1/1 -> add/2
  Zero_protection/1(r_out) -> Divide/2
  [r] -> Zero_protection/3(In3)
  Abs1/1 -> CompareToConstant1/1
  Subtract/1 -> Abs1/1
  MinMax/1 -> Subtract/2

== system KD_cl_harness_cl_ouports_added/ctrl_rb_explicit_20140220_v6_simp/HQPKWIK_V6/QPKWIK_Main/QPKWIK_While_Loop/Case3/full_step ==
  Primal : Inport
  c : Inport  Port=2
  Dual : Inport  Port=3
  b : Inport  Port=4
  SL_active_in : Inport  Port=5
  x_update : ActionPort  ActionType=then
  Add : Sum
  Gain : Gain  Gain=-1
  Gain1 : Gain
  Gain2 : Gain  OutDataTypeStr=int32
  Product : Product  Multiplication=Matrix(*)  RndMeth=Zero
  Product1 : Product  Multiplication=Matrix(*)  RndMeth=Zero
  Transpose : Math  Operator=transpose  SaturateOnIntegerOverflow=on
  x_out : Outport  InitialOutput=ov_zero_vec
  SL_active_out : Outport  Port=2  InitialOutput=0
  wires:
  SL_active_in/1 -> Gain2/1
  Gain2/1 -> SL_active_out/1
  Gain1/1 -> x_out/1
  Transpose/1 -> Product1/1
  Add/1 -> Gain1/1
  Product1/1 -> Add/2
  Product/1 -> Add/1
  b/1 -> Product1/2
  Dual/1 -> Transpose/1
  c/1 -> Product/2
  Gain/1 -> Product/1
  Primal/1 -> Gain/1

== system KD_cl_harness_cl_ouports_added/ctrl_rb_explicit_20140220_v6_simp/HQPKWIK_V6/QPKWIK_Main/QPKWIK_While_Loop/Case3/mid_step ==
  x_in : Inport
  t : Inport  Port=2
  z : Inport  Port=3
  SL_active_in : Inport  Port=4
  x_no_update : ActionPort  ActionType=elseif
  Add : Sum
  Gain1 : Gain
  Gain2 : Gain  OutDataTypeStr=int32
  Product : Product  RndMeth=Zero
  x_out : Outport  InitialOutput=ov_zero_vec
  SL_active_out : Outport  Port=2  InitialOutput=1
  wires:
  SL_active_in/1 -> Gain2/1
  Gain2/1 -> SL_active_out/1
  Add/1 -> Gain1/1
  Product/1 -> Add/2
  x_in/1 -> Add/1
  z/1 -> Product/2
  t/1 -> Product/1
  Gain1/1 -> x_out/1

== system KD_cl_harness_cl_ouports_added/ctrl_rb_explicit_20140220_v6_simp/HQPKWIK_V6/QPKWIK_Main/QPKWIK_While_Loop/Case3/no_update ==
  x_in : Inport
  x_no_update : ActionPort  ActionType=else
  Gain1 : Gain
  infeasible : Constant  Value=-1  OutDataTypeStr=int32
  x_out : Outport  InitialOutput=ov_zero_vec
  active_SL_infeas : Outport  Port=2  InitialOutput=-1
  wires:
  infeasible/1 -> active_SL_infeas/1
  x_in/1 -> Gain1/1
  Gain1/1 -> x_out/1

== system KD_cl_harness_cl_ouports_added/ctrl_rb_explicit_20140220_v6_simp/HQPKWIK_V6/QPKWIK_Main/QPKWIK_While_Loop/Case3/precomp_index ==
  S_L : Inport
  Abs : Abs  SaturateOnIntegerOverflow=on
  Active_set_equals_num_opt_variables : Subsystem  TreatAsAtomicUnit=on
  CompareToConstant : simulink/Logic and Bit Operations/Compare To Constant  relop=<=  const=0  OutDataTypeStr=boolean
  CompareToZero : simulink/Logic and Bit Operations/Compare To Zero  relop=>  OutDataTypeStr=boolean
  Constant3 : Constant  Value=ones_vec  VectorParams1D=off  OutDataTypeStr=uint32
      settings: AttributesFormatString=%<VectorParams1D>
  Data Type Conversion : DataTypeConversion  OutDataTypeStr=uint32
  DataTypeConversion{1..4} (4 alike) : DataTypeConversion  OutDataTypeStr=int32
  Extraction_of_Dual_and_Primal_matrices : Subsystem  TreatAsAtomicUnit=on
  Gain : Gain  OutDataTypeStr=int32
  If : If  NumInputs=2  IfExpression=u1==0  ElseIfExpressions=u1==u2
  Merge : Merge  Inputs=3
  Merge1 : Merge  Inputs=3
  Nominal_case : Subsystem  TreatAsAtomicUnit=on
  Product1 : Product  Multiplication=Matrix(*)  OutDataTypeStr=uint32  RndMeth=Zero
  Product11 : Product  Multiplication=Matrix(*)  OutDataTypeStr=int32  RndMeth=Zero
  Product8 : Product  Multiplication=Matrix(*)  OutDataTypeStr=uint32  RndMeth=Zero
  Subtract : Sum  Inputs=+-
  number_of_optimization_variables : Constant  Value=length_L  OutDataTypeStr=uint32
  one_to_vec_length : Constant  Value=one_to_vec_length  VectorParams1D=off
      settings: AttributesFormatString=%<Value>\n%<VectorParams1D>
  transpose{,1..3} (4 alike) : Math  Operator=transpose  SaturateOnIntegerOverflow=on
  vector_of_unique_ids : Constant  Value=vec  VectorParams1D=off
      settings: AttributesFormatString=%<Value>\n%<VectorParams1D>
  vector_of_unique_ids1 : Constant  Value=bin_vec  VectorParams1D=off
      settings: AttributesFormatString=%<Value>\n%<VectorParams1D>
  Primal_array : Outport
  Dual_array : Outport  Port=2
  Active_SL : Outport  Port=3
  wires:
  DataTypeConversion4/1 -> Subtract/1, Gain/1
  DataTypeConversion3/1 -> Product11/2
  DataTypeConversion2/1 -> Product11/1
  DataTypeConversion1/1 -> Subtract/2
  Product1/1 -> DataTypeConversion4/1
  [ind] -> Extraction_of_Dual_and_Primal_matrices/1(index)
  Product8/1 -> If/1
  Product11/1 -> [ind]
  Merge/1 -> Primal_array/1
  Merge1/1 -> Dual_array/1
  [ind] -> Active_set_equals_num_opt_variables/1(index)
  one_to_vec_length/1 -> transpose1/1
  Subtract/1 -> Abs/1
  Abs/1 -> CompareToConstant/1
  vector_of_unique_ids/1 -> transpose/1
  S_L/1 -> CompareToZero/1
  CompareToZero/1 -> Data Type Conversion/1
  Nominal_case/1(Primal_array) -> [Primal_A]
  Extraction_of_Dual_and_Primal_matrices/1(Primal_array) -> [Primal_C]
  Active_set_equals_num_opt_variables/1(Primal_array) -> [Primal_B]
  [Primal_A] -> Merge/1
  [Primal_B] -> Merge/2
  [Primal_C] -> Merge/3
  [Dual_A] -> Merge1/1
  [Dual_B] -> Merge1/2
  [Dual_C] -> Merge1/3
  Nominal_case/2(Dual_array) -> [Dual_A]
  Active_set_equals_num_opt_variables/2(Dual_array) -> [Dual_B]
  Extraction_of_Dual_and_Primal_matrices/2(Dual_array) -> [Dual_C]
  If/3 -> Extraction_of_Dual_and_Primal_matrices/Action
  If/2 -> Active_set_equals_num_opt_variables/Action
  If/1 -> Nominal_case/Action
  number_of_optimization_variables/1 -> If/2
  Data Type Conversion/1 -> transpose2/1, transpose3/1
  CompareToConstant/1 -> DataTypeConversion2/1
  transpose1/1 -> DataTypeConversion3/1
  transpose/1 -> DataTypeConversion1/1
  Gain/1 -> Active_SL/1
  transpose2/1 -> Product8/1
  Constant3/1 -> Product8/2
  transpose3/1 -> Product1/1
  vector_of_unique_ids1/1 -> Product1/2

== system KD_cl_harness_cl_ouports_added/ctrl_rb_explicit_20140220_v6_simp/HQPKWIK_V6/QPKWIK_Main/QPKWIK_While_Loop/Case3/t2 ==
  b : Inport
  A : Inport  Port=2
  knext : Inport  Port=3
  x : Inport  Port=4
  z : Inport  Port=5
  t2_calc : ActionPort  ActionType=else
  Add : Sum  Inputs=+-
  Add1 : Sum
  Divide : Product  Inputs=*/
  Divide_by_zero_protect : Subsystem
  Product : Product  Multiplication=Matrix(*)  RndMeth=Zero
  Product1 : Product  Multiplication=Matrix(*)  RndMeth=Zero
  Product2 : Product  RndMeth=Zero
  Product3 : Product  RndMeth=Zero
  extracts_ith_element_of_b : Selector  IndexOptions=Index vector (port)  Indices=[1:3]  OutputSizes=1
  extracts_ith_row_of_A : Selector  NumberOfDimensions=2  IndexOptions=Select all,Index vector (port)  Indices=[1:3],[1:3]  OutputSizes=1,1
  infinity : Constant  Value=HQP_INF  OutDataTypeStr=single
  transpose : Math  Operator=transpose  SaturateOnIntegerOverflow=on
  transpose1 : Math  Operator=transpose  SaturateOnIntegerOverflow=on
  t2 : Outport  InitialOutput=0
  wires:
  transpose/1 -> Product1/1
  extracts_ith_row_of_A/1 -> transpose1/1, Product1/2
  z/1 -> transpose/1
  Add/1 -> Divide/1
  Product/1 -> Add/2
  transpose1/1 -> Product/1
  x/1 -> Product/2
  extracts_ith_element_of_b/1 -> Add/1
  knext/1 -> extracts_ith_row_of_A/2, extracts_ith_element_of_b/2
  b/1 -> extracts_ith_element_of_b/1
  A/1 -> extracts_ith_row_of_A/1
  Product1/1 -> Divide_by_zero_protect/1(denom_in)
  Divide_by_zero_protect/1(denom_out) -> Divide/2
  infinity/1 -> Product2/2
  Product2/1 -> Add1/1
  Divide_by_zero_protect/2(zero) -> Product2/1
  Product3/1 -> Add1/2
  Add1/1 -> t2/1
  Divide_by_zero_protect/3(not_zero) -> Product3/1
  Divide/1 -> [t2_temp]
  [t2_temp] -> Product3/2

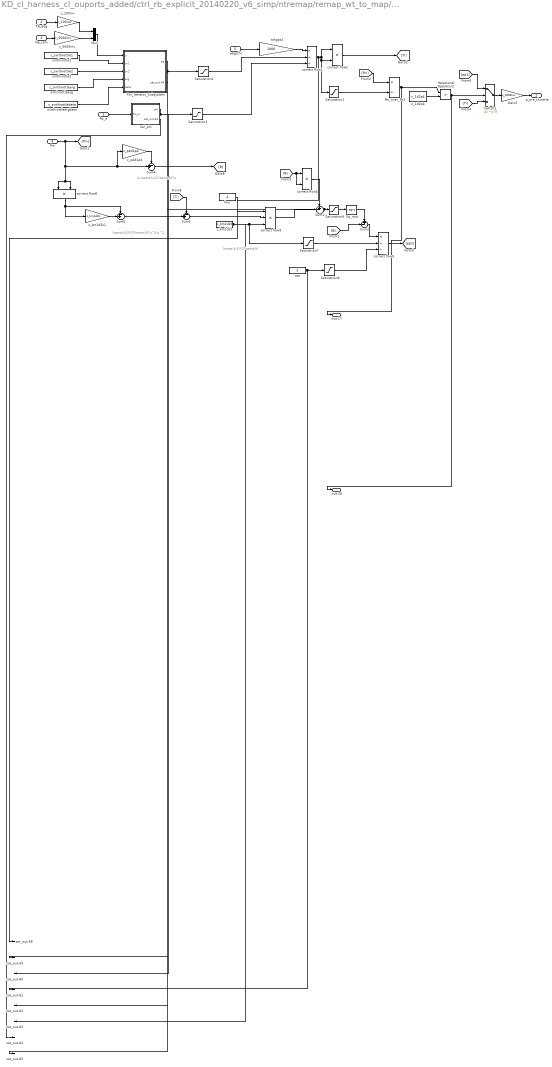
== system KD_cl_harness_cl_ouports_added/ctrl_rb_explicit_20140220_v6_simp/ntremap/remap_wt_to_map/ThrottleModel1/AirModel_map_use/Forward_Flow ==
  note: (const.k-1)/(2*const.k)
  note: (const.k-1)/(2*const.k)*u^2-u^2
  note: u-(const.k-1)/(const.k)*u
  Ro_a : Inport
  TA_deg : Inport  Port=2
  Ne_rpm : Inport  Port=3
  Pm : Inport  Port=4
  wegrthr : Inport  Port=5
  Cal_phi : Subsystem
  For_Iterator_Subsystem : Subsystem  TreatAsAtomicUnit=on
  Gain2 : Gain  Gain=c_1000inv
  Mux : Mux  Inputs=2
  Pm_over_Pa2 : Product  Inputs=*/  SaturateOnIntegerOverflow=on  RndMeth=Zero  InputSameDT=on  OutDataTypeStr=Inherit: Same as first input
  Relational Operator2 : RelationalOperator  Operator=>  OutDataTypeStr=boolean
      settings: AttributesFormatString=%<Operator>
  Saturation{1..4,7} (5 alike) : Saturate  UpperLimit=c_inf  LowerLimit=c_p1e9
      settings: AttributesFormatString=%<LowerLimit>\n%<UpperLimit>
  Saturation6 : Saturate  UpperLimit=inf  LowerLimit=0
      settings: AttributesFormatString=%<LowerLimit>\n%<UpperLimit>
  Sq_root : Sqrt  AlgorithmType=Newton-Raphson  SaturateOnIntegerOverflow=on
  Sum1 : Sum  Inputs=+-|
  Sum2 : Sum  Inputs=+-|
  Sum3 : Sum  Inputs=-+|
  Sum4 : Sum  Inputs=-+|
  Sum5 : Sum  Inputs=-+|
  Switch2 : Switch  Criteria=u2 ~= 0
      settings: AttributesFormatString=%<Criteria>
  c_100inv : Gain  Gain=c_100inv
  c_1d2p4 : Constant  Value=c_1d2p4  OutDataTypeStr=single  SampleTime=-1
      settings: AttributesFormatString=%<Value>\n%<SampleTime>
  c_5500inv : Gain  Gain=c_5500inv
  c_km1d2k : Constant  Value=c_km1d2k  OutDataTypeStr=single  SampleTime=-1
      settings: AttributesFormatString=%<Value>\n%<SampleTime>
  c_km1d2k1 : Gain  Gain=c_km1d2k
  c_p4d1p4 : Gain  Gain=c_p4d1p4
  correct flow1 : Product  Inputs=*//  SaturateOnIntegerOverflow=on  RndMeth=Zero  InputSameDT=on  OutDataTypeStr=Inherit: Same as first input
  correct flow2 : Product  Inputs=**  SaturateOnIntegerOverflow=on  RndMeth=Zero  InputSameDT=on  OutDataTypeStr=Inherit: Same as first input
  correct flow3 : Product  Inputs=***  SaturateOnIntegerOverflow=on  RndMeth=Zero  InputSameDT=on  OutDataTypeStr=Inherit: Same as first input
  correct flow4 : Product  Inputs=**  SaturateOnIntegerOverflow=on  RndMeth=Zero  InputSameDT=on  OutDataTypeStr=Inherit: Same as first input
  correct flow5 : Product  Inputs=*//  SaturateOnIntegerOverflow=on  RndMeth=Zero  InputSameDT=on  OutDataTypeStr=Inherit: Same as first input
  correct flow6 : Product  Inputs=**  SaturateOnIntegerOverflow=on  RndMeth=Zero  InputSameDT=on  OutDataTypeStr=Inherit: Same as first input
  four : Constant  Value=4  OutDataTypeStr=single  SampleTime=-1
      settings: AttributesFormatString=%<Value>\n%<SampleTime>
  svrthrottle1 : Constant  Value=c_svrthrottle1  OutDataTypeStr=single  SampleTime=-1
      settings: AttributesFormatString=%<Value>\n%<SampleTime>
  svrthrottle2 : Constant  Value=c_svrthrottle2  OutDataTypeStr=single  SampleTime=-1
      settings: AttributesFormatString=%<Value>\n%<SampleTime>
  svrthrottlearg : Constant  Value=c_svrthrottlearg  OutDataTypeStr=single  SampleTime=-1
      settings: AttributesFormatString=%<Value>\n%<SampleTime>
  svrthrottleargbeta : Constant  Value=c_svrthrottlebeta  OutDataTypeStr=single  SampleTime=-1
      settings: AttributesFormatString=%<Value>\n%<SampleTime>
  tokgps2 : Gain  Gain=1000
  two : Constant  Value=2  OutDataTypeStr=single  SampleTime=-1
      settings: AttributesFormatString=%<Value>\n%<SampleTime>
  p_pre_throttle : Outport  OutDataTypeStr=single
  sat_out-58 : Outport  Port=2
  sat_out-59 : Outport  Port=3
  sat_out-60 : Outport  Port=4
  sat_out-61 : Outport  Port=5
  sat_out-62 : Outport  Port=6
  sat_out-63 : Outport  Port=7
  sat_out-64 : Outport  Port=8
  sat_out-65 : Outport  Port=9
  out-17 : Outport  Port=10
  out-28 : Outport  Port=11
  wires:
  c_km1d2k1/1 -> Sum5/2
  c_p4d1p4/1 -> Sum4/1
  Relational Operator2/1 -> Switch2/2, out-28/1
  Pm_over_Pa2/1 -> Relational Operator2/1, out-17/1
  c_1d2p4/1 -> Relational Operator2/2
  correct flow6/1 -> Sum5/1, c_km1d2k1/1
  Sum5/1 -> Sum3/2
  svrthrottleargbeta/1 -> For_Iterator_Subsystem/5(beta)
  svrthrottlearg/1 -> For_Iterator_Subsystem/4(arg)
  svrthrottle2/1 -> For_Iterator_Subsystem/3(sv2)
  svrthrottle1/1 -> For_Iterator_Subsystem/2(sv1)
  Saturation6/1 -> Sq_root/1
  Sum3/1 -> correct flow3/2
  [pp1] -> Switch2/1
  correct flow5/1 -> [pp1]
  [Ti] -> Sum3/1
  [Ti] -> Switch2/3
  correct flow2/1 -> [Ti]
  [Pin] -> Pm_over_Pa2/1
  [B] -> Sum2/2
  [B] -> correct flow4/2, correct flow4/1
  Sum4/1 -> [B]
  For_Iterator_Subsystem/1(ba) -> Saturation2/1, sat_out-59/1
  Saturation4/1 -> correct flow5/3
  Saturation7/1 -> correct flow5/2
  Saturation3/1 -> correct flow1/3
  Saturation2/1 -> correct flow1/2
  Saturation1/1 -> Pm_over_Pa2/2
  correct flow4/1 -> Sum1/1
  Gain2/1 -> p_pre_throttle/1
  Switch2/1 -> Gain2/1
  two/1 -> Saturation4/1, sat_out-61/1
  Sum2/1 -> correct flow5/1
  Sq_root/1 -> Sum2/1
  Sum1/1 -> Saturation6/1, sat_out-62/1
  correct flow3/1 -> Sum1/2
  c_km1d2k/1 -> Saturation7/1, correct flow3/3, sat_out-63/1
  four/1 -> correct flow3/1
  correct flow1/1 -> Saturation1/1, correct flow2/2, correct flow2/1, sat_out-58/1
  tokgps2/1 -> correct flow1/1
  wegrthr/1 -> tokgps2/1
  Ne_rpm/1 -> c_5500inv/1
  c_5500inv/1 -> Mux/2
  c_100inv/1 -> Mux/1
  TA_deg/1 -> c_100inv/1
  Mux/1 -> For_Iterator_Subsystem/1(u)
  Ro_a/1 -> Cal_phi/1(Ro_a)
  Pm/1 -> [Pin], correct flow6/2, correct flow6/1, c_p4d1p4/1, Sum4/2
  Cal_phi/1(phi) -> Saturation3/1, sat_out-60/1
  Cal_phi/2(sat_out-64) -> sat_out-64/1
  For_Iterator_Subsystem/2(sat_out-65) -> sat_out-65/1

== system KD_cl_harness_cl_ouports_added/ctrl_rb_explicit_20140220_v6_simp/HQPKWIK_V6/QPKWIK_Main/QPKWIK_While_Loop/Case3/Dual_and_Primal_step/step_is_t1 ==
  n_act : Inport
  constraints_vec : Inport  Port=2
  S_L : Inport  Port=3
  mu : Inport  Port=4
  kdrop : Inport  Port=5
  step_is_t2 : ActionPort  ActionType=else
  Abs : Abs  SaturateOnIntegerOverflow=on
  CompareToZero : simulink/Logic and Bit Operations/Compare To Zero  relop=>  OutDataTypeStr=boolean
  DataTypeConversion1 : DataTypeConversion  OutDataTypeStr=int32
  DataTypeConversion2 : DataTypeConversion  OutDataTypeStr=single
  Gain : Gain  OutDataTypeStr=int32
  Product1 : Product  OutDataTypeStr=int32  RndMeth=Zero
  Product2 : Product  RndMeth=Zero
  Subtract : Sum  Inputs=+-
  add : Sum  OutDataTypeStr=int32
  case : Constant  Value=2  OutDataTypeStr=uint8
  reduce_num_constraints : Constant  Value=-1  OutDataTypeStr=int32
  n_act_out : Outport  InitialOutput=0
  Case : Outport  Port=2  InitialOutput=2
  S_L_out : Outport  Port=3  InitialOutput=zero_vec
  mu_out : Outport  Port=4  InitialOutput=zero_vec
  wires:
  DataTypeConversion2/1 -> Product2/1
  DataTypeConversion1/1 -> Product1/1
  Gain/1 -> S_L_out/1
  constraints_vec/1 -> Subtract/2
  kdrop/1 -> Subtract/1
  Product2/1 -> mu_out/1
  mu/1 -> Product2/2
  reduce_num_constraints/1 -> add/1
  n_act/1 -> add/2
  add/1 -> n_act_out/1
  case/1 -> Case/1
  S_L/1 -> Product1/2
  Product1/1 -> Gain/1
  Subtract/1 -> Abs/1
  Abs/1 -> CompareToZero/1
  CompareToZero/1 -> DataTypeConversion2/1, DataTypeConversion1/1

== system KD_cl_harness_cl_ouports_added/ctrl_rb_explicit_20140220_v6_simp/HQPKWIK_V6/QPKWIK_Main/QPKWIK_While_Loop/Case3/Dual_and_Primal_step/step_is_t2 ==
  n_act : Inport
  input : Inport  Port=2
  k_next : Inport  Port=3
  S_L : Inport  Port=4
  mu : Inport  Port=5
  step_is_t1 : ActionPort  ActionType=then
  DataTypeConversion1 : DataTypeConversion  OutDataTypeStr=int32
  Gain : Gain  OutDataTypeStr=int32
  Product1 : Product  OutDataTypeStr=int32  RndMeth=Zero
  RelationalOperator : RelationalOperator  Operator=~=  OutDataTypeStr=boolean
  add : Sum  OutDataTypeStr=int32
  add1 : Sum
  case : Constant  OutDataTypeStr=uint8
  increase_number_active : Constant  OutDataTypeStr=int32
  true : Constant  OutDataTypeStr=boolean
  n_act_out : Outport  InitialOutput=0
  Case : Outport  Port=2  InitialOutput=1
  S_L_out : Outport  Port=3  InitialOutput=zero_vec
  mu_out : Outport  Port=4  InitialOutput=zero_vec
  wires:
  DataTypeConversion1/1 -> Product1/1
  Gain/1 -> S_L_out/1
  add1/1 -> Gain/1
  Product1/1 -> add1/1
  mu/1 -> mu_out/1
  S_L/1 -> add1/2
  k_next/1 -> Product1/2
  input/1 -> RelationalOperator/1
  true/1 -> RelationalOperator/2
  case/1 -> Case/1
  add/1 -> n_act_out/1
  n_act/1 -> add/2
  increase_number_active/1 -> add/1
  RelationalOperator/1 -> DataTypeConversion1/1

== system KD_cl_harness_cl_ouports_added/ctrl_rb_explicit_20140220_v6_simp/HQPKWIK_V6/QPKWIK_Main/QPKWIK_While_Loop/Case3/T1_calculation/Zero_protection ==
  In2 : Inport
  In1 : Inport  Port=2
  In3 : Inport  Port=3
  CompareToZero : simulink/Logic and Bit Operations/Compare To Zero  relop=<=  OutDataTypeStr=boolean
  DataTypeConversion1 : DataTypeConversion  OutDataTypeStr=single
  Infinity : Constant  Value=HQP_INF  OutDataTypeStr=single
  Product : Product  RndMeth=Zero
  Product3 : Product  RndMeth=Zero
  add : Sum
  r_out : Outport
  wires:
  DataTypeConversion1/1 -> Product/1
  In1/1 -> CompareToZero/1
  In2/1 -> Product3/2
  Product3/1 -> add/1
  Product/1 -> add/2
  Infinity/1 -> Product/2
  add/1 -> r_out/1
  CompareToZero/1 -> DataTypeConversion1/1
  In3/1 -> Product3/1

== system KD_cl_harness_cl_ouports_added/ctrl_rb_explicit_20140220_v6_simp/HQPKWIK_V6/QPKWIK_Main/QPKWIK_While_Loop/Case3/precomp_index/Active_set_equals_num_opt_variables ==
  index : Inport
  Active_set_equals_numb_opt_variables : ActionPort  ActionType=elseif
  DataTypeConversion1 : DataTypeConversion  OutDataTypeStr=int32
  Dual_Array : Constant  Value=Dual_array  OutDataTypeStr=single
  Gain : Gain  Gain=0
  MinMax : MinMax  Inputs=2
  extracts_ith_page_of_array : Selector  NumberOfDimensions=3  IndexOptions=Select all,Select all,Index vector (port)  Indices=[1:10],[1:3],[1:3]  OutputSizes=1,1,1
  size_Dual : Constant  Value=size_dual  OutDataTypeStr=single
  zero_primal_matrix : Constant  Value=L2  OutDataTypeStr=single
  Primal_array : Outport  InitialOutput=primal_init
  Dual_array : Outport  Port=2  InitialOutput=dual_zero
  wires:
  DataTypeConversion1/1 -> MinMax/2
  size_Dual/1 -> DataTypeConversion1/1
  MinMax/1 -> extracts_ith_page_of_array/2
  index/1 -> MinMax/1
  Gain/1 -> Primal_array/1
  zero_primal_matrix/1 -> Gain/1
  extracts_ith_page_of_array/1 -> Dual_array/1
  Dual_Array/1 -> extracts_ith_page_of_array/1

== system KD_cl_harness_cl_ouports_added/ctrl_rb_explicit_20140220_v6_simp/HQPKWIK_V6/QPKWIK_Main/QPKWIK_While_Loop/Case3/precomp_index/Extraction_of_Dual_and_Primal_matrices ==
  index : Inport
  Extraction_of_Dual_and_Primal_Matrices : ActionPort  ActionType=else
  DataTypeConversion1 : DataTypeConversion  OutDataTypeStr=int32
  DataTypeConversion2 : DataTypeConversion  OutDataTypeStr=int32
  Dual_Array : Constant  Value=Dual_array  OutDataTypeStr=single
  MinMax : MinMax  Inputs=2
  MinMax1 : MinMax  Inputs=2
  Primal_Array : Constant  Value=Primal_array  OutDataTypeStr=single
  extracts_ith_page_of_array : Selector  NumberOfDimensions=3  IndexOptions=Select all,Select all,Index vector (port)  Indices=[1:3],[1:3],[1:3]  OutputSizes=1,1,1
  extracts_ith_page_of_array1 : Selector  NumberOfDimensions=3  IndexOptions=Select all,Select all,Index vector (port)  Indices=[1:10],[1:3],[1:3]  OutputSizes=1,1,1
  size_Dua : Constant  Value=size_dual  OutDataTypeStr=single
  size_Primal : Constant  Value=size_primal  OutDataTypeStr=single
  Primal_array : Outport  InitialOutput=primal_init
  Dual_array : Outport  Port=2  InitialOutput=dual_zero
  wires:
  DataTypeConversion2/1 -> MinMax1/2
  DataTypeConversion1/1 -> MinMax/2
  MinMax1/1 -> extracts_ith_page_of_array1/2
  size_Dua/1 -> DataTypeConversion2/1
  MinMax/1 -> extracts_ith_page_of_array/2
  index/1 -> MinMax1/1, MinMax/1
  size_Primal/1 -> DataTypeConversion1/1
  extracts_ith_page_of_array1/1 -> Dual_array/1
  extracts_ith_page_of_array/1 -> Primal_array/1
  Dual_Array/1 -> extracts_ith_page_of_array1/1
  Primal_Array/1 -> extracts_ith_page_of_array/1

== system KD_cl_harness_cl_ouports_added/ctrl_rb_explicit_20140220_v6_simp/HQPKWIK_V6/QPKWIK_Main/QPKWIK_While_Loop/Case3/precomp_index/Nominal_case ==
  Nominal_case : ActionPort  ActionType=then
  Dual_Array : Constant  Value=Dual_array  OutDataTypeStr=single
  Primal_Array : Constant  Value=Primal_array  OutDataTypeStr=single
  extracts_ith_page_of_array : Selector  NumberOfDimensions=3  IndexOptions=Select all,Select all,Index vector (port)  Indices=[1:3],[1:3],[1:3]  OutputSizes=1,1,1
  extracts_ith_page_of_array1 : Selector  NumberOfDimensions=3  IndexOptions=Select all,Select all,Index vector (port)  Indices=[1:num_constraints],[1:3],[1:3]  OutputSizes=1,1,1
  size_dual : Constant  Value=size_dual  OutDataTypeStr=single
  size_primal : Constant  Value=size_primal  OutDataTypeStr=single
  Primal_array : Outport  InitialOutput=primal_init
  Dual_array : Outport  Port=2  InitialOutput=dual_zero
  wires:
  size_dual/1 -> extracts_ith_page_of_array1/2
  size_primal/1 -> extracts_ith_page_of_array/2
  extracts_ith_page_of_array1/1 -> Dual_array/1
  extracts_ith_page_of_array/1 -> Primal_array/1
  Dual_Array/1 -> extracts_ith_page_of_array1/1
  Primal_Array/1 -> extracts_ith_page_of_array/1

== system KD_cl_harness_cl_ouports_added/ctrl_rb_explicit_20140220_v6_simp/HQPKWIK_V6/QPKWIK_Main/QPKWIK_While_Loop/Case3/t2/Divide_by_zero_protect ==
  denom_in : Inport
  Absolute_value : Abs
  Add1 : Sum
  DataTypeConversion1 : DataTypeConversion  OutDataTypeStr=single
  DataTypeConversion2 : DataTypeConversion  OutDataTypeStr=single
  Product2 : Product  RndMeth=Zero
  Product3 : Product  RndMeth=Zero
  RelationalOperator : RelationalOperator  Operator=<=  OutDataTypeStr=boolean
  RelationalOperator1 : RelationalOperator  Operator=>  OutDataTypeStr=boolean
  epsilon : Constant  Value=HQP_eps  OutDataTypeStr=single
  epsilon1 : Constant  Value=HQP_eps  OutDataTypeStr=single
  epsilon2 : Constant  Value=HQP_eps  OutDataTypeStr=single
  denom_out : Outport
  zero : Outport  Port=2
  not_zero : Outport  Port=3
  wires:
  DataTypeConversion2/1 -> zero/1, Product2/1
  DataTypeConversion1/1 -> not_zero/1, Product3/1
  epsilon1/1 -> RelationalOperator/2
  denom_in/1 -> Product3/2, Absolute_value/1
  Absolute_value/1 -> RelationalOperator1/1, RelationalOperator/1
  epsilon/1 -> RelationalOperator1/2
  epsilon2/1 -> Product2/2
  Product2/1 -> Add1/1
  RelationalOperator/1 -> DataTypeConversion2/1
  Product3/1 -> Add1/2
  RelationalOperator1/1 -> DataTypeConversion1/1
  Add1/1 -> denom_out/1

== system KD_cl_harness_cl_ouports_added/ctrl_rb_explicit_20140220_v6_simp/ntremap/remap_wt_to_map/ThrottleModel1/AirModel_map_use/Forward_Flow/Cal_phi ==
  Ro_a : Inport
  Gain2 : Gain  Gain=c_roacorr  SaturateOnIntegerOverflow=on  OutDataTypeStr=Inherit: Same as input  ParamDataTypeStr=Inherit: Same as input
  Saturation6 : Saturate  UpperLimit=inf  LowerLimit=0
      settings: AttributesFormatString=%<LowerLimit>\n%<UpperLimit>
  Sqrt : Sqrt  AlgorithmType=Newton-Raphson  SaturateOnIntegerOverflow=on
  phi : Outport
  sat_out-64 : Outport  Port=2
  wires:
  Saturation6/1 -> Sqrt/1
  Gain2/1 -> Saturation6/1, sat_out-64/1
  Ro_a/1 -> Gain2/1
  Sqrt/1 -> phi/1
